simulink model "joint_sim"  (R2018b)
settings: Solver=FixedStepAuto  StartTime=0.0  StopTime=3  FixedStep=0.001  MaxStep=0.001  RelTol=1e-3
values from neighbouring files (symbols this model uses):
  alpha = 1.0    (= 1)    [init.m]
  D_el = 0    [init.m]
  F_c = 35    [init.m]
  F_s = 40    [init.m]
  J_joint = 4.155    [init.m]
  J_load = 1.2252    [init.m]
  K_el = 6900    [init.m]
  Kd_pos = 410.747040    (= 410.74704)    [init.m]
  Kd_trq = 0    [init.m]
  Kp_pos = 6124.290039    [init.m]
  Kp_trq = 0    [init.m]
  Ks_pos = 0.006793    [init.m]
  Ks_trq = 0.04    [init.m]
  Kt_pos = 0.126640    (= 0.12664)    [init.m]
  Kt_trq = 9.10251    [init.m]
  sigma0 = 2000    [init.m]
  sigma1 = 200    [init.m]
  sigma2 = D_visc    (= 20)    [init.m]
  T_cur = 2e-3    (= 0.002)    [init.m]
  T_signal_LPF = 2e-3    (= 0.002)    [init.m]
  tau_max_ctrl = 180    [init.m]
  vs = 0.1    [init.m]
undefined symbols (not defined in the file or in its folder): X, Y, Z
libraries: sm_lib x6, nesl_utility x3, fcnLib4joint_sim x2, simulink x2
settings Model: Creator=l.ho  LastModifiedBy=qiming

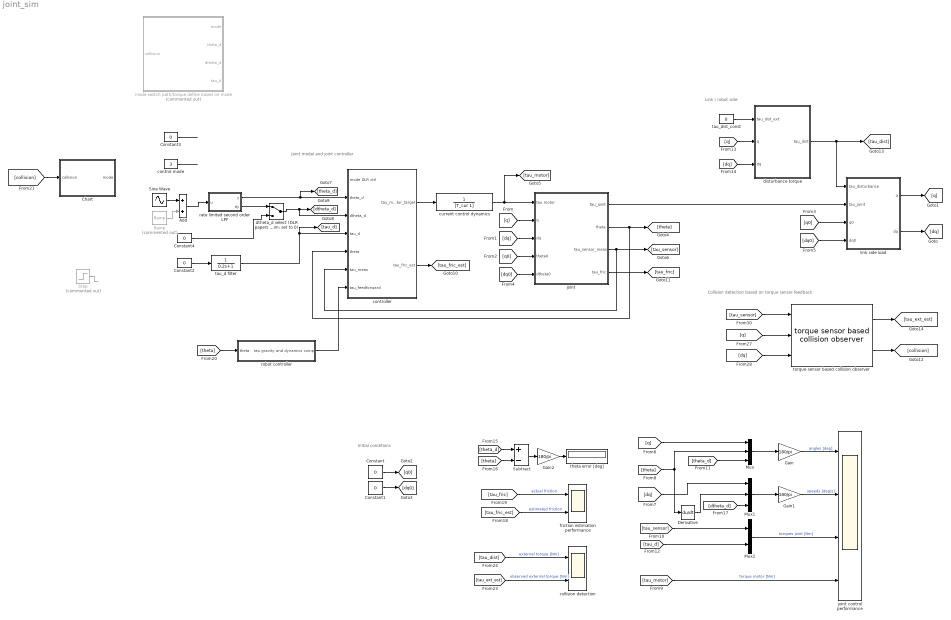
== system joint_sim ==
  note: Collision detection based on torque sensor feedback
  note: Initial conditions
  note: Joint model and joint controller
  note: Link / robot side
  " torque sensor based collision observer " : fcnLib4joint_sim/ torque sensor based collision observer   SystemSampleTime=-1
  Add : Sum
  Chart : Stateflow chart  TreatAsAtomicUnit=on
  Constant{,1..4} (5 alike) : Constant  Value=0
  Derivative : Derivative
  Gain : Gain  Gain=180/pi
  Gain1 : Gain  Gain=180/pi
  Gain2 : Gain  Gain=180/pi
  Mux : Mux  Inputs=3
  Mux1 : Mux  Inputs=3
  Mux2 : Mux  Inputs=2
  Ramp : simulink/Sources/Ramp  Commented=on  slope=0.2  start=0.5  InitialOutput=0
  Sine Wave : Sin  Frequency=pi/3  SampleTime=0
  Step : Step  Commented=on  Time=0.1  After=0.1  SampleTime=0
  Subtract : Sum  Inputs=+-
  "collision detection " : Scope  NumInputPorts=2
  control mode : Constant  Value=3
  controller : Subsystem
  current control dynamics : TransferFcn  Denominator=[T_cur 1]
  disturbance torque : Subsystem
  dtheta_d select (DLR papers and sim: set to 0) : ManualSwitch
  friction estimation performance : Scope  NumInputPorts=2
  joint : Subsystem
  joint control performance : Scope  NumInputPorts=4
  link side load : Subsystem
  mode switch path/torque define based on mode : Subsystem  Commented=on
  rate limited second order LPF : Subsystem
  robot controller : Subsystem
  tau_d filter : TransferFcn  Denominator=[0.2 1]
  tau_dist_const : Constant  Value=0
  theta error [deg] : Display
  wires:
  Constant/1 -> [q0]
  Constant1/1 -> [dq0]
  controller/1(tau_motor_target) -> current control dynamics/1
  joint/1(tau_joint) -> link side load/2(tau_joint)
  [dq0] -> link side load/4(dq0)
  [q0] -> link side load/3(q0)
  link side load/2(dq) -> [dq]
  link side load/1(q) -> [q]
  joint/2(theta) -> [theta], controller/5(theta)
  joint/3(tau_sensor_meas) -> controller/6(tau_meas), [tau_sensor]
  tau_dist_const/1 -> disturbance torque/1(tau_dist_ext)
  disturbance torque/1(tau_dist) -> [tau_dist], link side load/1(tau_disturbance)
  current control dynamics/1 -> [tau_motor], joint/1(tau motor)
  Constant2/1 -> tau_d filter/1
  [theta] -> Mux/2, Derivative/1
  [q] -> Mux/1
  Mux/1 -> Gain/1
  Mux1/1 -> Gain1/1
  [dq] -> Mux1/1
  Derivative/1 -> Mux1/2
  [tau_sensor] -> Mux2/1
  Mux2/1 -> joint control performance/3  "torques joint [Nm]"
  Add/1 -> rate limited second order LPF/1(u)
  [theta_d] -> Mux/3
  [tau_d] -> Mux2/2
  rate limited second order LPF/1(y) -> [theta_d], controller/2(theta_d)
  tau_d filter/1 -> [tau_d], controller/4(tau_d)
  [q] -> disturbance torque/2(q)
  [dq] -> disturbance torque/3(dq)
  Gain/1 -> joint control performance/1  "angles [deg]"
  Gain1/1 -> joint control performance/2  "speeds [deg/s]"
  [theta_d] -> Subtract/1
  [theta] -> Subtract/2
  Subtract/1 -> Gain2/1
  Gain2/1 -> theta error [deg]/1
  dtheta_d select (DLR papers and sim: set to 0)/1 -> controller/3(dtheta_d), [dtheta_d]
  [dtheta_d] -> Mux1/3
  controller/2(tau_fric_est) -> [tau_fric_est]
  joint/4(tau_fric) -> [tau_fric]
  [tau_fric] -> friction estimation performance/1  "actual friction"
  [tau_fric_est] -> friction estimation performance/2  "estimated friction"
  [tau_motor] -> joint control performance/4  "torque motor [Nm]"
  [theta] -> robot controller/1(theta)
  robot controller/1(tau gravity and dynamics comp.) -> controller/7(tau_feedforward)
  rate limited second order LPF/2(dy) -> dtheta_d select (DLR papers and sim: set to 0)/1
  Constant4/1 -> dtheta_d select (DLR papers and sim: set to 0)/2
  Step/1 -> ?
  Ramp/1 -> Add/2
  [tau_ext_est] -> "collision detection "/2  "observed external torque [Nm]"
  [tau_dist] -> "collision detection "/1  "external torque [Nm]"
  [dq0] -> joint/5(dtheta0)
  [q] -> joint/2(q)
  [q0] -> joint/4(theta0)
  [dq] -> joint/3(dq)
  [q] -> " torque sensor based collision observer "/2
  " torque sensor based collision observer "/1 -> [tau_ext_est]
  [tau_sensor] -> " torque sensor based collision observer "/1
  [dq] -> " torque sensor based collision observer "/3
  " torque sensor based collision observer "/2 -> [collision]
  Sine Wave/1 -> Add/1
  Constant3/1 -> ?
  control mode/1 -> ?
  ? -> controller/1(mode DLR ctrl)
  [collision] -> Chart/1(collision)

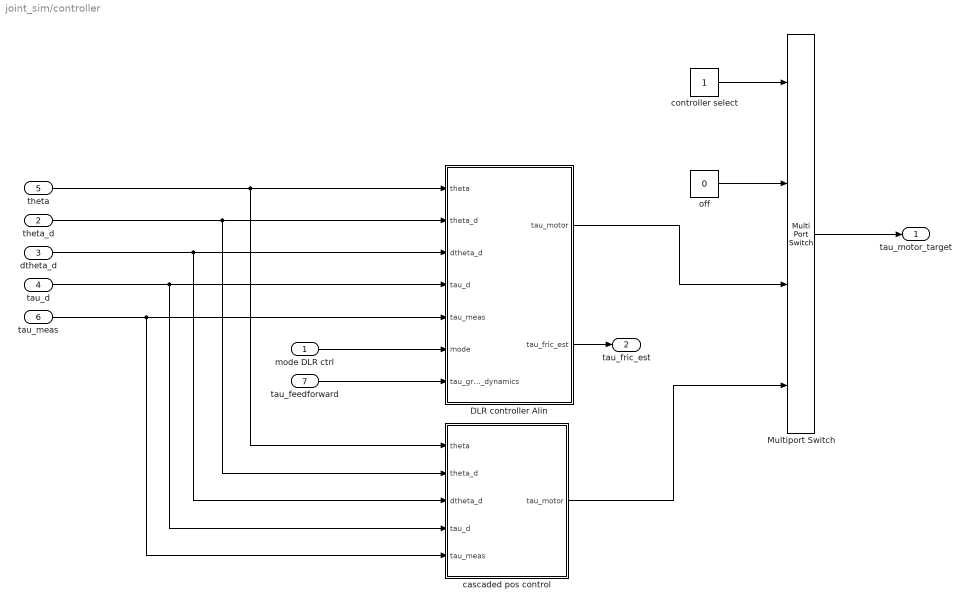
== system joint_sim/controller ==
  mode DLR ctrl : Inport
  theta_d : Inport  Port=2
  dtheta_d : Inport  Port=3
  tau_d : Inport  Port=4
  theta : Inport  Port=5
  tau_meas : Inport  Port=6
  tau_feedforward : Inport  Port=7
  DLR controller Alin : Subsystem
  Multiport Switch : MultiPortSwitch  DataPortOrder=Zero-based contiguous  zeroidx=on
  cascaded pos control : Subsystem
  controller select : Constant
  off : Constant  Value=0
  tau_motor_target : Outport
  tau_fric_est : Outport  Port=2
  wires:
  Multiport Switch/1 -> tau_motor_target/1
  off/1 -> Multiport Switch/2
  controller select/1 -> Multiport Switch/1
  cascaded pos control/1(tau_motor) -> Multiport Switch/4
  theta/1 -> cascaded pos control/1(theta), DLR controller Alin/1(theta)
  theta_d/1 -> cascaded pos control/2(theta_d), DLR controller Alin/2(theta_d)
  tau_d/1 -> cascaded pos control/4(tau_d), DLR controller Alin/4(tau_d)
  DLR controller Alin/1(tau_motor) -> Multiport Switch/3
  mode DLR ctrl/1 -> DLR controller Alin/6(mode)
  tau_meas/1 -> DLR controller Alin/5(tau_meas), cascaded pos control/5(tau_meas)
  dtheta_d/1 -> cascaded pos control/3(dtheta_d), DLR controller Alin/3(dtheta_d)
  DLR controller Alin/2(tau_fric_est) -> tau_fric_est/1
  tau_feedforward/1 -> DLR controller Alin/7(tau_gravity_and_dynamics)

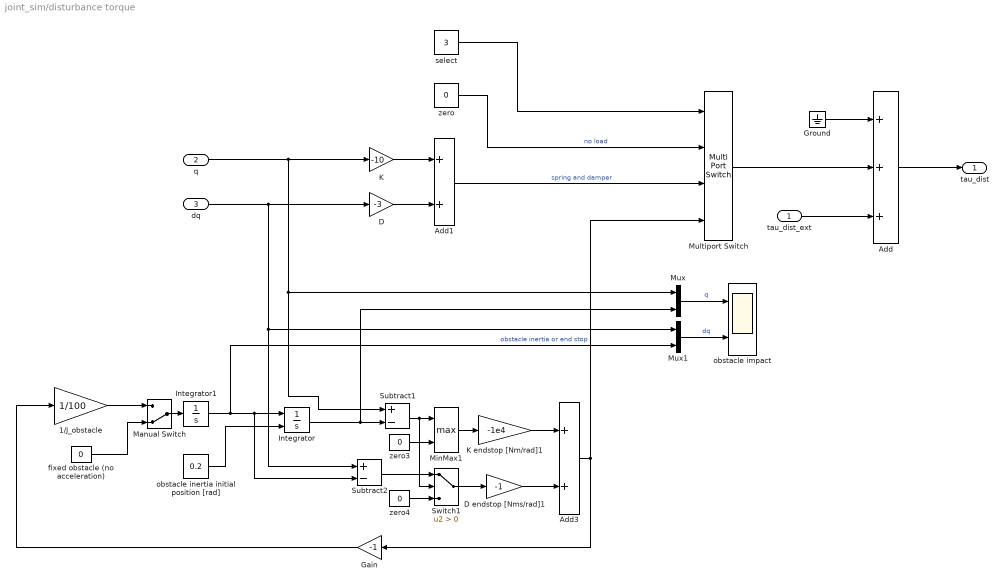
== system joint_sim/disturbance torque ==
  tau_dist_ext : Inport
  q : Inport  Port=2
  dq : Inport  Port=3
  1/J_obstacle : Gain  Gain=1/100
  Add : Sum  Inputs=+++
  Add1 : Sum
  Add3 : Sum
  D : Gain  Gain=-3
  D endstop [Nms/rad]1 : Gain  Gain=-1
  Gain : Gain  Gain=-1
  Ground : Ground
  Integrator : Integrator  InitialConditionSource=external
  Integrator1 : Integrator
  K : Gain  Gain=-10
  K endstop [Nm/rad]1 : Gain  Gain=-1e4
  Manual Switch : ManualSwitch  CurrentSetting=0
  MinMax1 : MinMax  Function=max  Inputs=2
  Multiport Switch : MultiPortSwitch
  Mux : Mux  Inputs=2
  Mux1 : Mux  Inputs=2
  Subtract1 : Sum  Inputs=+-
  Subtract2 : Sum  Inputs=+-
  Switch1 : Switch  Criteria=u2 > Threshold
  fixed obstacle (no acceleration) : Constant  Value=0
  obstacle impact : Scope  NumInputPorts=2
  obstacle inertia initial position [rad] : Constant  Value=0.2
  select : Constant  Value=3
  zero : Constant  Value=0
  zero3 : Constant  Value=0
  zero4 : Constant  Value=0
  tau_dist : Outport
  wires:
  Add/1 -> tau_dist/1
  tau_dist_ext/1 -> Add/3
  Ground/1 -> Add/1
  Add1/1 -> Multiport Switch/3  "spring and damper"
  K/1 -> Add1/1
  D/1 -> Add1/2
  Multiport Switch/1 -> Add/2
  zero/1 -> Multiport Switch/2  "no load"
  select/1 -> Multiport Switch/1
  dq/1 -> D/1, Mux1/1, Subtract2/1
  zero4/1 -> Switch1/3
  D endstop [Nms/rad]1/1 -> Add3/2
  Switch1/1 -> D endstop [Nms/rad]1/1
  zero3/1 -> MinMax1/2
  MinMax1/1 -> K endstop [Nm/rad]1/1
  K endstop [Nm/rad]1/1 -> Add3/1
  Subtract1/1 -> MinMax1/1, Switch1/2
  Integrator/1 -> Mux/2, Subtract1/2
  Integrator1/1 -> Mux1/2, Subtract2/2, Integrator/1
  obstacle inertia initial position [rad]/1 -> Integrator/2
  Add3/1 -> Gain/1, Multiport Switch/4  "obstacle inertia or end stop"
  Gain/1 -> 1/J_obstacle/1
  Subtract2/1 -> Switch1/1
  q/1 -> Mux/1, Subtract1/1, K/1
  Mux/1 -> obstacle impact/1  "q"
  Mux1/1 -> obstacle impact/2  "dq"
  Manual Switch/1 -> Integrator1/1
  1/J_obstacle/1 -> Manual Switch/1
  fixed obstacle (no acceleration)/1 -> Manual Switch/2

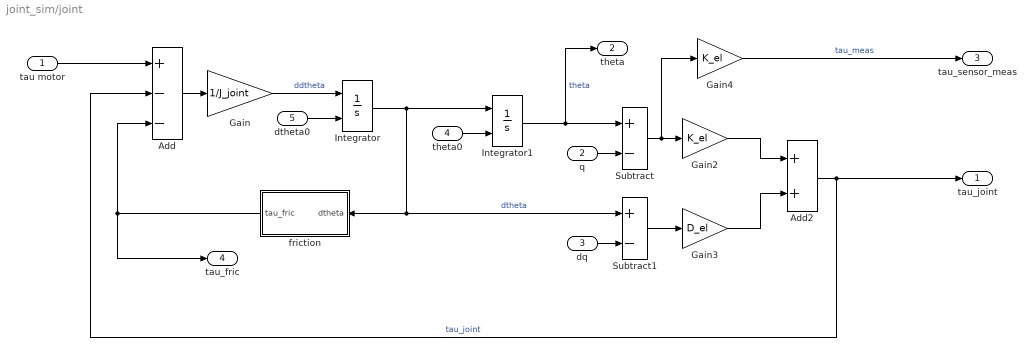
== system joint_sim/joint ==
  tau motor : Inport
  q : Inport  Port=2
  dq : Inport  Port=3
  theta0 : Inport  Port=4
  dtheta0 : Inport  Port=5
  Add : Sum  Inputs=+--
  Add2 : Sum
  Gain : Gain  Gain=1/J_joint
  Gain2 : Gain  Gain=K_el
  Gain3 : Gain  Gain=D_el
  Gain4 : Gain  Gain=K_el
  Integrator : Integrator  InitialConditionSource=external
  Integrator1 : Integrator  InitialConditionSource=external
  Subtract : Sum  Inputs=+-
  Subtract1 : Sum  Inputs=+-
  friction : Subsystem
  tau_joint : Outport
  theta : Outport  Port=2
  tau_sensor_meas : Outport  Port=3
  tau_fric : Outport  Port=4
  wires:
  q/1 -> Subtract/2
  Gain4/1 -> tau_sensor_meas/1  "tau_meas"
  Gain/1 -> Integrator/1  "ddtheta"
  Gain3/1 -> Add2/2
  Gain2/1 -> Add2/1
  Add2/1 -> tau_joint/1, Add/2  "tau_joint"
  theta0/1 -> Integrator1/2
  Integrator/1 -> Integrator1/1, Subtract1/1, friction/1(dtheta)  "dtheta"
  Subtract/1 -> Gain4/1, Gain2/1
  Subtract1/1 -> Gain3/1
  tau motor/1 -> Add/1
  Add/1 -> Gain/1
  Integrator1/1 -> theta/1, Subtract/1  "theta"
  dtheta0/1 -> Integrator/2
  friction/1(tau_fric) -> tau_fric/1, Add/3
  dq/1 -> Subtract1/2

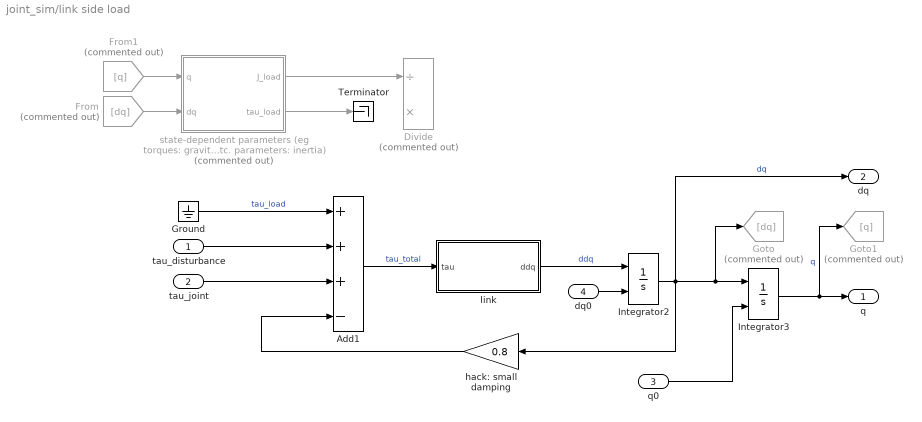
== system joint_sim/link side load ==
  tau_disturbance : Inport
  tau_joint : Inport  Port=2
  q0 : Inport  Port=3
  dq0 : Inport  Port=4
  Add1 : Sum  Inputs=+++-
  Divide : Product  Commented=on  Inputs=/*
  From : From  Commented=on  GotoTag=dq
  From1 : From  Commented=on  GotoTag=q
  Goto : Goto  Commented=on  GotoTag=dq
  Goto1 : Goto  Commented=on  GotoTag=q
  Ground : Ground
  Integrator2 : Integrator  InitialConditionSource=external
  Integrator3 : Integrator  InitialConditionSource=external
  Terminator : Terminator
  hack: small damping : Gain  Gain=0.8
  link : Subsystem
  "state-dependent parameters (eg torques: gravity, Coriolis, etc. parameters: inertia)" : Subsystem  Commented=on
  q : Outport
  dq : Outport  Port=2
  wires:
  tau_joint/1 -> Add1/3
  Integrator2/1 -> hack: small damping/1, dq/1, Goto/1, Integrator3/1  "dq"
  q0/1 -> Integrator3/2
  link/1(ddq) -> Integrator2/1  "ddq"
  tau_disturbance/1 -> Add1/2
  Add1/1 -> link/1(tau)  "tau_total"
  Integrator3/1 -> Goto1/1, q/1  "q"
  dq0/1 -> Integrator2/2
  "state-dependent parameters (eg torques: gravity, Coriolis, etc. parameters: inertia)"/2(tau_load) -> Terminator/1
  From/1 -> "state-dependent parameters (eg torques: gravity, Coriolis, etc. parameters: inertia)"/2(dq)
  From1/1 -> "state-dependent parameters (eg torques: gravity, Coriolis, etc. parameters: inertia)"/1(q)
  "state-dependent parameters (eg torques: gravity, Coriolis, etc. parameters: inertia)"/1(J_load) -> Divide/1
  hack: small damping/1 -> Add1/4
  Ground/1 -> Add1/1  "tau_load"

== system joint_sim/mode switch path//torque define based on mode ==
  note: control mode:
      | 0 = zero_force
      | 1 = torque
      | 2 = impedance
      | 3 = position
  collision : Inport
  Constant3 : Constant  Value=0
  Switch : Switch  Criteria=u2 ~= 0
  control mode : Constant  Value=3
  mode : Outport
  theta_d : Outport  Port=2
  dtheta_d : Outport  Port=3
  tau_d : Outport  Port=4
  wires:
  Switch/1 -> ?
  control mode/1 -> Switch/3
  Constant3/1 -> Switch/1
  collision/1 -> ?

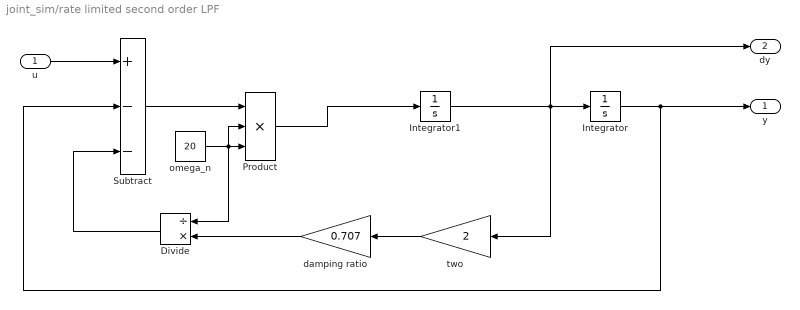
== system joint_sim/rate limited second order LPF ==
  u : Inport
  Divide : Product  Inputs=/*
  Integrator : Integrator
  Integrator1 : Integrator  LimitOutput=on  UpperSaturationLimit=1  LowerSaturationLimit=-1
  Product : Product  Inputs=3
  Subtract : Sum  Inputs=+--
  damping ratio : Gain  Gain=0.707
  omega_n : Constant  Value=20
  two : Gain  Gain=2
  y : Outport
  dy : Outport  Port=2
  wires:
  Integrator1/1 -> two/1, dy/1, Integrator/1
  Integrator/1 -> Subtract/2, y/1
  u/1 -> Subtract/1
  Subtract/1 -> Product/1
  Product/1 -> Integrator1/1
  two/1 -> damping ratio/1
  Divide/1 -> Subtract/3
  omega_n/1 -> Divide/1, Product/2, Product/3
  damping ratio/1 -> Divide/2

== system joint_sim/robot controller ==
  note: input list is still incomplete
  theta : Inport
  Ground : Ground
  Terminator : Terminator
  tau gravity and dynamics comp. : Outport
  wires:
  Ground/1 -> tau gravity and dynamics comp./1
  theta/1 -> Terminator/1

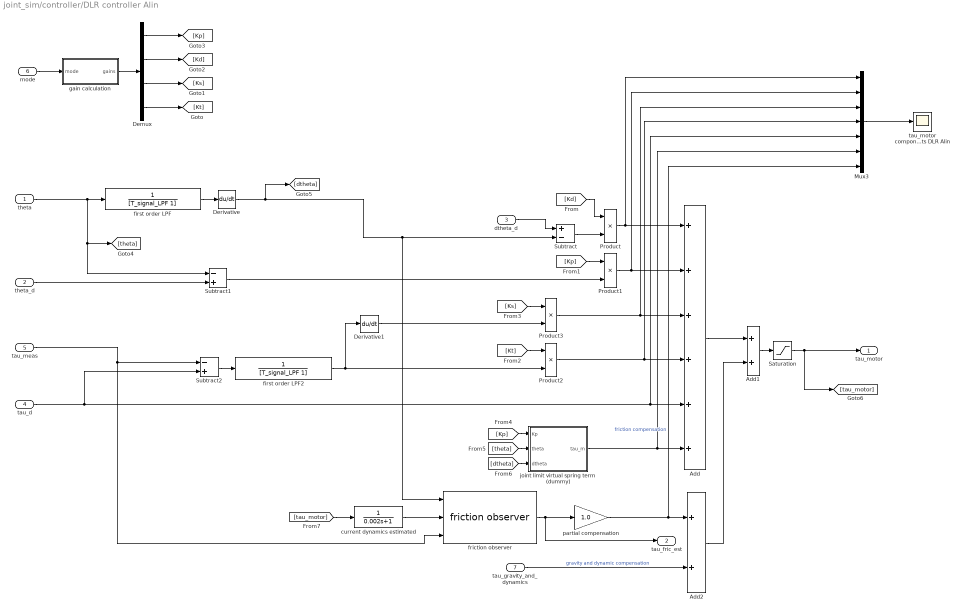
== system joint_sim/controller/DLR controller Alin ==
  theta : Inport
  theta_d : Inport  Port=2
  dtheta_d : Inport  Port=3
  tau_d : Inport  Port=4
  tau_meas : Inport  Port=5
  mode : Inport  Port=6
  tau_gravity_and_dynamics : Inport  Port=7
  Add : Sum  Inputs=++++++
  Add1 : Sum
  Add2 : Sum
  Demux : Demux
  Derivative : Derivative
  Derivative1 : Derivative
  Mux3 : Mux  Inputs=7
  Product{,1..3} (4 alike) : Product
  Saturation : Saturate  UpperLimit=tau_max_ctrl  LowerLimit=-tau_max_ctrl  LinearizeAsGain=off  ZeroCross=off
  Subtract : Sum  Inputs=+-
  Subtract1 : Sum  Inputs=-+
  Subtract2 : Sum  Inputs=-+
  current dynamics estimated : TransferFcn  Denominator=[0.002 1]
  first order LPF : TransferFcn  Denominator=[T_signal_LPF 1]
  first order LPF2 : TransferFcn  Denominator=[T_signal_LPF 1]
  friction observer : fcnLib4joint_sim/friction observer  SystemSampleTime=-1
  gain calculation : Subsystem
  joint limit virtual spring term (dummy) : Subsystem
  partial compensation : Gain  Gain=1.0
  tau_motor components DLR Alin : Scope
  tau_motor : Outport
  tau_fric_est : Outport  Port=2
  wires:
  Derivative1/1 -> Product3/2
  first order LPF2/1 -> Product2/2, Derivative1/1
  Product2/1 -> Mux3/4, Add/4
  Subtract/1 -> Product/2
  [Ks] -> Product3/1
  theta/1 -> [theta], Subtract1/1, first order LPF/1
  Add2/1 -> Add1/2
  partial compensation/1 -> Mux3/7, Add2/1  "friction compensation"
  Product/1 -> Mux3/1, Add/1
  joint limit virtual spring term (dummy)/1(tau_m) -> Mux3/6, Add/6
  tau_gravity_and_dynamics/1 -> Add2/2  "gravity and dynamic compensation"
  Product3/1 -> Mux3/3, Add/3
  first order LPF/1 -> Derivative/1
  Derivative/1 -> [dtheta], friction observer/1, Subtract/2
  [Kd] -> Product/1
  Saturation/1 -> [tau_motor], tau_motor/1
  dtheta_d/1 -> Subtract/1
  tau_d/1 -> Mux3/5, Add/5, Subtract2/2
  [Kp] -> joint limit virtual spring term (dummy)/1(Kp)
  Mux3/1 -> tau_motor components DLR Alin/1
  Product1/1 -> Mux3/2, Add/2
  Add/1 -> Add1/1
  [theta] -> joint limit virtual spring term (dummy)/2(theta)
  Subtract1/1 -> Product1/2
  Subtract2/1 -> first order LPF2/1
  [dtheta] -> joint limit virtual spring term (dummy)/3(dtheta)
  Add1/1 -> Saturation/1
  [Kt] -> Product2/1
  [Kp] -> Product1/1
  theta_d/1 -> Subtract1/2
  Demux/4 -> [Kt]
  Demux/2 -> [Kd]
  Demux/1 -> [Kp]
  Demux/3 -> [Ks]
  mode/1 -> gain calculation/1(mode)
  gain calculation/1(gains) -> Demux/1
  [tau_motor] -> current dynamics estimated/1
  current dynamics estimated/1 -> friction observer/2
  tau_meas/1 -> friction observer/3, Subtract2/1
  friction observer/1 -> tau_fric_est/1, partial compensation/1

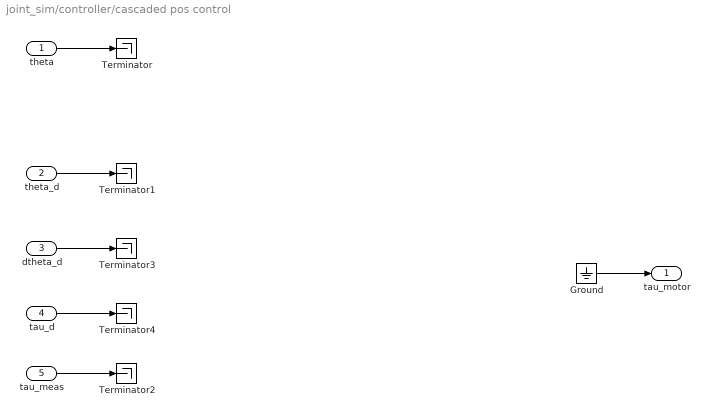
== system joint_sim/controller/cascaded pos control ==
  theta : Inport
  theta_d : Inport  Port=2
  dtheta_d : Inport  Port=3
  tau_d : Inport  Port=4
  tau_meas : Inport  Port=5
  Ground : Ground
  Terminator{,1..4} (5 alike) : Terminator
  tau_motor : Outport
  wires:
  theta/1 -> Terminator/1
  theta_d/1 -> Terminator1/1
  tau_meas/1 -> Terminator2/1
  Ground/1 -> tau_motor/1
  dtheta_d/1 -> Terminator3/1
  tau_d/1 -> Terminator4/1

== system joint_sim/joint/friction ==
  dtheta : Inport
  Add : Sum
  Compare To Constant : simulink/Logic and Bit Operations/Compare To Constant  relop=>=  const=0.01  OutDataTypeStr=boolean
  Constant : Constant  Value=F_c
  Gain4 : Gain  Gain=sigma2
  Subsystem : Subsystem
  tau_fric : Outport
  wires:
  dtheta/1 -> Subsystem/1(v), Gain4/1
  Gain4/1 -> Add/1  "viscous friction"
  Add/1 -> tau_fric/1
  Constant/1 -> Compare To Constant/1
  Compare To Constant/1 -> Subsystem/Enable
  Subsystem/1(F_fric dynamic) -> Add/2  "dynamic Stribeck friction"

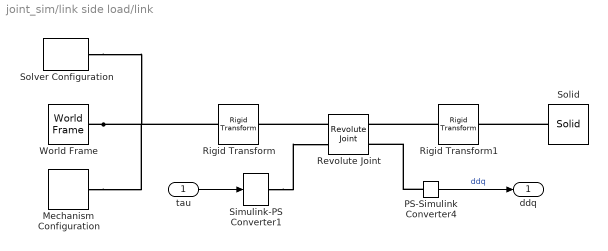
== system joint_sim/link side load/link ==
  tau : Inport
  Mechanism Configuration : sm_lib/Utilities/Mechanism Configuration  UniformGravity=Constant  GravityVector=[0 0 -9.80665]  GravityUnits=m/s^2  LinearizationDelta=0.001
  PS-Simulink Converter4 : nesl_utility/PS-Simulink Converter  PhysicalDomain=network_engine_domain  SubClassName=ps_output  LeftPortType=input  RightPortType=output  PseudoPeriodic=off  Frequencies=[]  Unit=1  AffineConversion=off
  Revolute Joint : sm_lib/Joints/Revolute Joint  SenseConstraintForce=off  SenseConstraintForceX=off  SenseConstraintForceY=off  SenseConstraintForceZ=off  SenseConstraintTorque=off  SenseConstraintTorqueX=off  SenseConstraintTorqueY=off  SenseConstraintTorqueZ=off  SenseTotalForce=off  SenseTotalForceX=off  SenseTotalForceY=off  SenseTotalForceZ=off  SenseTotalTorque=off  SenseTotalTorqueX=off  SenseTotalTorqueY=off  SenseTotalTorqueZ=off  CompositeWrenchDir=FollowerOnBase  CompositeWrenchFrame=BaseFrame  EquilibriumPosition=0  EquilibriumPositionUnits=deg  SpringStiffness=0  SpringStiffnessUnits=N*m/deg  DampingCoefficient=0  DampingCoefficientUnits=N*m/(deg/s)  TorqueActuationMode=InputTorque  MotionActuationMode=ComputedMotion  SensePosition=off  SenseVelocity=off  SenseAcceleration=on  SenseTorqueForce=off  PositionTargetSpecify=off  PositionTargetPriority=High  PositionTargetValue=0  PositionTargetValueUnits=deg  VelocityTargetSpecify=off  VelocityTargetPriority=High  VelocityTargetValue=0  VelocityTargetValueUnits=deg/s
  Rigid Transform : sm_lib/Frames and Transforms/Rigid Transform  TranslationMethod=None  TranslationStandardOffset=150  TranslationLengthUnit=mm  TranslationStandardAxis=-X  TranslationCartesianOffset=[-150 0 0]  TranslationROffset=0  TranslationROffsetUnits=m  TranslationZOffset=0  TranslationZOffsetUnits=m  TranslationThetaOffset=0  TranslationThetaOffsetUnits=deg  RotationMethod=None  RotationAngleUnits=deg  RotationStandardAxis=+Z  RotationAngle=0.0  RotationArbitraryAxis=[0 0 1]  FollAlignAxisA=+X  BaseAlignAxisA=+Y  FollAlignAxisB=+Y  BaseAlignAxisB=+Z  RotationSequenceAxes=FollowerAxes  RotationSequence=XYX  RotationSequenceAngles=[0 0 0]  RotationSequenceAnglesUnits=deg  RotationMatrix=[1 0 0; 0 1 0; 0 0 1]
  Rigid Transform1 : sm_lib/Frames and Transforms/Rigid Transform  TranslationMethod=StandardAxis  TranslationStandardOffset=150  TranslationLengthUnit=mm  TranslationStandardAxis=+X  TranslationCartesianOffset=[0 0 0]  TranslationROffset=0  TranslationROffsetUnits=m  TranslationZOffset=0  TranslationZOffsetUnits=m  TranslationThetaOffset=0  TranslationThetaOffsetUnits=deg  RotationMethod=None  RotationAngleUnits=deg  RotationStandardAxis=+Z  RotationAngle=0.0  RotationArbitraryAxis=[0 0 1]  FollAlignAxisA=+X  BaseAlignAxisA=+Y  FollAlignAxisB=+Y  BaseAlignAxisB=+Z  RotationSequenceAxes=FollowerAxes  RotationSequence=XYX  RotationSequenceAngles=[0 0 0]  RotationSequenceAnglesUnits=deg  RotationMatrix=[1 0 0; 0 1 0; 0 0 1]
  Simulink-PS Converter1 : nesl_utility/Simulink-PS Converter  PhysicalDomain=network_engine_domain  SubClassName=ps_input  LeftPortType=input  RightPortType=output  PseudoPeriodic=off  Frequencies=[]  NoiseDistribution=none  NoiseParameters=[]  Unit=1  AffineConversion=off  FilteringAndDerivatives=provide  SimscapeFilterOrder=1  InputFilterTimeConstant=0.001  UdotUserProvided=0
  Solid : sm_lib/Body Elements/Solid  InertiaType=Custom  Mass=1  MassUnits=kg  CenterOfMass=[0 0 0]  CenterOfMassUnits=m  MomentsOfInertia=[1 1 1.2252]  MomentsOfInertiaUnits=kg*m^2  ProductsOfInertia=[0 0 0]  ProductsOfInertiaUnits=kg*m^2  BasedOnType=Density  Density=2700  DensityUnits=kg/m^3  DoExposeReferenceFrame=on  SerializedFrames=<Frames/>  GraphicType=FromGeometry  MarkerShape=Sphere  MarkerSize=10  GraphicVisPropType=SimpleVisualProperties  GraphicDiffuseColor=[0.5 0.5 0.5]  GraphicSpecularColor=[0.5 0.5 0.5 1.0]  GraphicAmbientColor=[0.15 0.15 0.15 1.0]  GraphicEmissiveColor=[0.0 0.0 0.0 1.0]  GraphicShininess=75  GraphicOpacity=1.0  GeometryShape=Brick  RectangleSize=[1 1]  RectangleSizeUnits=m  BrickDimensions=[300 30 30]  BrickDimensionUnits=mm  CylinderRadius=1  CylinderRadiusUnits=m  CylinderLength=1  CylinderLengthUnits=m  SphereRadius=1  SphereRadiusUnits=m  EllipsoidRadii=[1 1 1]  EllipsoidRadiiUnits=m  ExtrusionCrossSection=[1 1; -1 1; -1 -1; 1 -1]  ExtrusionCrossSectionUnits=m  ExtrusionLength=1  ExtrusionLengthUnits=m  PolygonNumSides=3  PolygonOuterRadius=1  PolygonOuterRadiusUnits=m  ExtGeomFileType=STEP  ExtGeomFileUnits=m  RevolutionCrossSection=[1 1; 1 -1; 2 -1; 2 1]  RevolutionCrossSectionUnits=m  RevolutionExtent=Full  RevolutionAngle=180  RevolutionAngleUnits=deg
  Solver Configuration : nesl_utility/Solver Configuration  PhysicalDomain=network_engine_domain  SubClassName=solver  LeftPortType=input  RightPortType=generic  Tones=[]  Harmonics=[]  SimulateNoise=off  Profile=off  UseLocalSampling=off  EnableSwitchedLinearOptims=on  FrequencyDomain=off  UseCCode=off  RelTol=0.001  AbsTol=1e-06  MinStep=1e-09  ToWorkspace=off  RevertToSquareIcSolve=off  NumHomotopyIterations=100  PhasorMode=off  PhasorModeNumHarmonics=1  DoDC=off  ResidualTolerance=1e-09  UseLocalSolver=off  LocalSolverChoice=NE_BACKWARD_EULER_ADVANCER  LocalSolverSampleTime=0.001  DoFixedCost=off  MaxNonlinIter=3  MaxModeIter=2  LinearAlgebra=auto  EquationFormulation=NE_TIME_EF  DelaysMemoryBudget=1024  AutomaticFiltering=on  FilteringTimeConstant=0.001  PartitionStorageMethod=AS_NEEDED  PartitionMemoryBudget=1024
  World Frame : sm_lib/Frames and Transforms/World Frame
  ddq : Outport
  wires:
  tau/1 -> Simulink-PS Converter1/1
  PS-Simulink Converter4/1 -> ddq/1  "ddq"
  connections:
  World Frame/RConn1 -- Rigid Transform/LConn1 -- Solver Configuration/RConn1 -- Mechanism Configuration/RConn1
  Simulink-PS Converter1/RConn1 -- Revolute Joint/LConn2
  Revolute Joint/LConn1 -- Rigid Transform/RConn1
  Solid/RConn1 -- Rigid Transform1/RConn1
  PS-Simulink Converter4/LConn1 -- Revolute Joint/RConn2
  Rigid Transform1/LConn1 -- Revolute Joint/RConn1

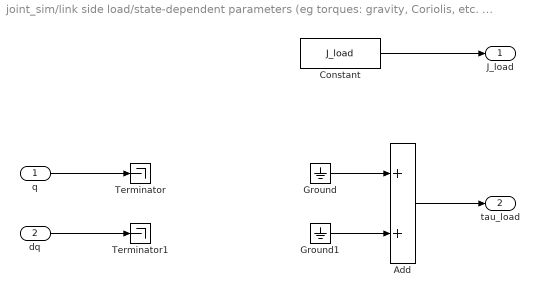
== system joint_sim/link side load/state-dependent parameters (eg torques: gravity, Coriolis, etc. parameters: inertia) ==
  q : Inport
  dq : Inport  Port=2
  Add : Sum
  Constant : Constant  Value=J_load
  Ground : Ground
  Ground1 : Ground
  Terminator : Terminator
  Terminator1 : Terminator
  J_load : Outport
  tau_load : Outport  Port=2
  wires:
  Add/1 -> tau_load/1
  q/1 -> Terminator/1
  dq/1 -> Terminator1/1
  Ground/1 -> Add/1
  Ground1/1 -> Add/2
  Constant/1 -> J_load/1

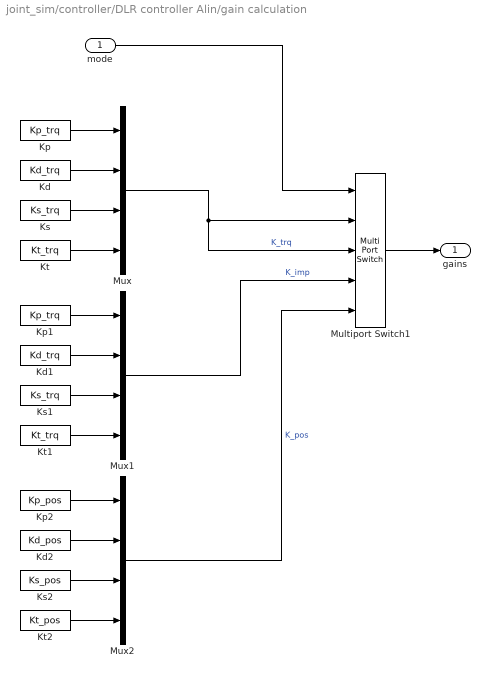
== system joint_sim/controller/DLR controller Alin/gain calculation ==
  mode : Inport
  Kd : Constant  Value=Kd_trq
  Kd1 : Constant  Value=Kd_trq
  Kd2 : Constant  Value=Kd_pos
  Kp : Constant  Value=Kp_trq
  Kp1 : Constant  Value=Kp_trq
  Kp2 : Constant  Value=Kp_pos
  Ks : Constant  Value=Ks_trq
  Ks1 : Constant  Value=Ks_trq
  Ks2 : Constant  Value=Ks_pos
  Kt : Constant  Value=Kt_trq
  Kt1 : Constant  Value=Kt_trq
  Kt2 : Constant  Value=Kt_pos
  Multiport Switch1 : MultiPortSwitch  DataPortOrder=Zero-based contiguous  Inputs=4  DiagnosticForDefault=None  zeroidx=on
  Mux : Mux
  Mux1 : Mux
  Mux2 : Mux
  gains : Outport
  wires:
  Mux/1 -> Multiport Switch1/2, Multiport Switch1/3  "K_trq"
  Kt1/1 -> Mux1/4
  Kd2/1 -> Mux2/2
  mode/1 -> Multiport Switch1/1
  Mux1/1 -> Multiport Switch1/4  "K_imp"
  Kp1/1 -> Mux1/1
  Kt2/1 -> Mux2/4
  Kp/1 -> Mux/1
  Kt/1 -> Mux/4
  Mux2/1 -> Multiport Switch1/5  "K_pos"
  Kd1/1 -> Mux1/2
  Ks2/1 -> Mux2/3
  Kd/1 -> Mux/2
  Ks1/1 -> Mux1/3
  Ks/1 -> Mux/3
  Kp2/1 -> Mux2/1
  Multiport Switch1/1 -> gains/1

== system joint_sim/controller/DLR controller Alin/joint limit virtual spring term (dummy) ==
  Kp : Inport
  theta : Inport  Port=2
  dtheta : Inport  Port=3
  Ground : Ground
  Terminator : Terminator
  Terminator1 : Terminator
  Terminator2 : Terminator
  tau_m : Outport
  wires:
  Ground/1 -> tau_m/1
  dtheta/1 -> Terminator2/1
  Kp/1 -> Terminator/1
  theta/1 -> Terminator1/1

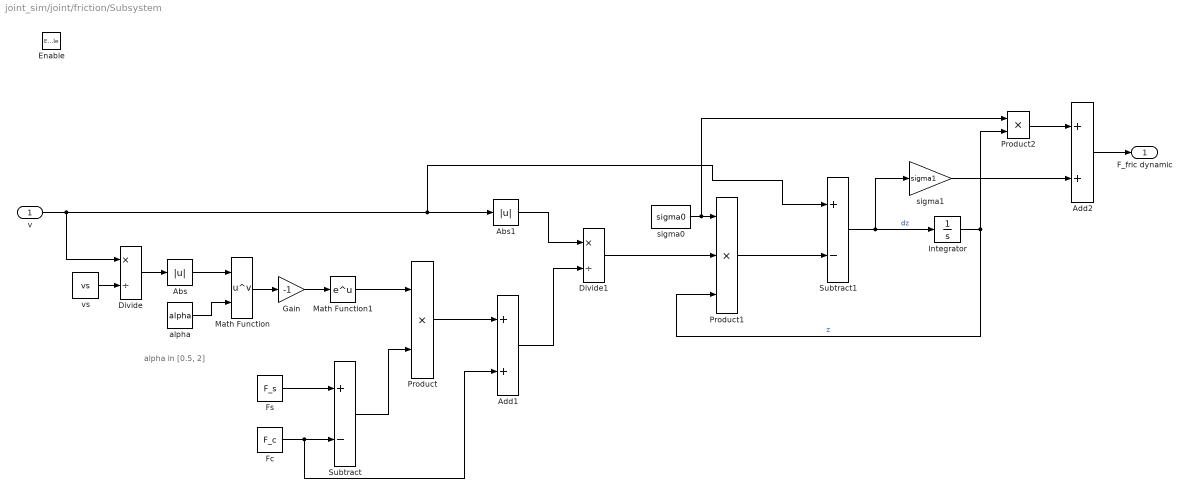
== system joint_sim/joint/friction/Subsystem ==
  note: alpha in [0.5, 2]
  v : Inport
  Enable : EnablePort  StatesWhenEnabling=reset
  Abs : Abs
  Abs1 : Abs
  Add1 : Sum
  Add2 : Sum
  Divide : Product  Inputs=*/
  Divide1 : Product  Inputs=*/
  Fc : Constant  Value=F_c
  Fs : Constant  Value=F_s
  Gain : Gain  Gain=-1
  Integrator : Integrator
  Math Function : Math  Operator=pow  SaturateOnIntegerOverflow=on
  Math Function1 : Math  SaturateOnIntegerOverflow=on
  Product : Product
  Product1 : Product  Inputs=3
  Product2 : Product
  Subtract : Sum  Inputs=+-
  Subtract1 : Sum  Inputs=+-
  alpha : Constant  Value=alpha
  sigma0 : Constant  Value=sigma0
  sigma1 : Gain  Gain=sigma1
  vs : Constant  Value=vs
  F_fric dynamic : Outport  OutputWhenDisabled=reset  InitialOutput=0
  wires:
  Product1/1 -> Subtract1/2
  Divide1/1 -> Product1/2
  Abs/1 -> Math Function/1
  sigma1/1 -> Add2/2
  sigma0/1 -> Product2/1, Product1/1
  v/1 -> Subtract1/1, Abs1/1, Divide/1
  Product2/1 -> Add2/1
  Product/1 -> Add1/1
  Subtract/1 -> Product/2
  Math Function1/1 -> Product/1
  Divide/1 -> Abs/1
  alpha/1 -> Math Function/2
  Integrator/1 -> Product2/2, Product1/3  "z"
  Gain/1 -> Math Function1/1
  Fc/1 -> Add1/2, Subtract/2
  vs/1 -> Divide/2
  Subtract1/1 -> sigma1/1, Integrator/1  "dz"
  Math Function/1 -> Gain/1
  Add1/1 -> Divide1/2
  Abs1/1 -> Divide1/1
  Fs/1 -> Subtract/1
  Add2/1 -> F_fric dynamic/1

== stateflow chart joint_sim/Chart ==
  data: collision input; mode output
